simulink library "Power_Ideal2Motor"  (R2020a)
settings: Solver=VariableStepAuto  StartTime=0.0  StopTime=10.0  RelTol=1e-3
undefined symbols (not defined in the file): ShaftF, ShaftR
libraries: fl_lib x11, nesl_utility x6, sm_lib x1
Description:
  | Component of Simscape Vehicle Templates Library
  | 
  | Copyright 2018-2020 The MathWorks, Inc.
settings Model: Creator=smiller  LastModifiedBy=smiller
settings DataIOCC: ReturnWorkspaceOutputs=off
settings DebuggingCC: ArithmeticOperatorsInVariantConditions=warning
settings SFSimCC: CustomCodeUndefinedFunction=UseInterfaceOnly

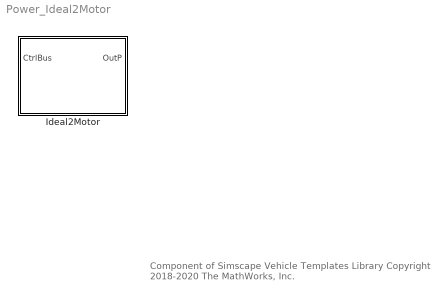
== system Power_Ideal2Motor ==
  note: Component of Simscape Vehicle Templates Library
      | Copyright 2018-2020 The MathWorks, Inc.
  Ideal2Motor : Subsystem  VariantControl=IdealTwoMotor  mask(Two Ideal Motors){motor_ts_f=100, motor_ts_r=100}
      mask prompts: motor_ts_f "Front Motor Cutoff Frequency (Hz)"; motor_ts_r "Rear Motor Cutoff Frequency (Hz)"
      mask Display: image('sm_car_vehicle_power_ideal2motor_IMAGE.png');

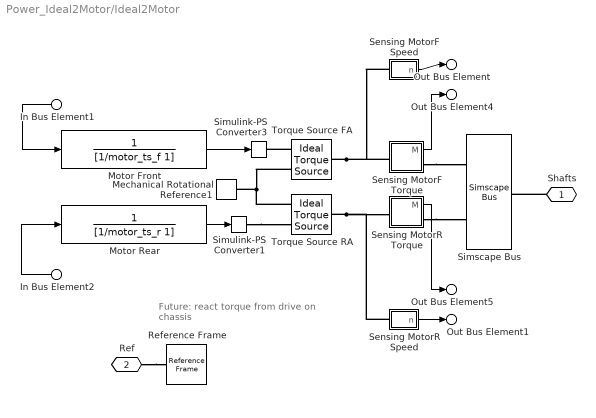
== system Power_Ideal2Motor/Ideal2Motor ==
  note: Future: react torque from
      | drive on chassis
  In Bus Element1 : Inport  PortName=CtrlBus  Element=MMotorFDemand
  In Bus Element2 : Inport  PortName=CtrlBus  Element=MMotorRDemand
  Mechanical Rotational Reference1 : fl_lib/Mechanical/Rotational Elements/Mechanical Rotational Reference
  Motor Front : TransferFcn  Denominator=[1/motor_ts_f 1]
  Motor Rear : TransferFcn  Denominator=[1/motor_ts_r 1]
  Reference Frame : sm_lib/Frames and Transforms/Reference Frame
  Sensing MotorF Speed : Subsystem
  Sensing MotorF Torque : Subsystem
  Sensing MotorR Speed : Subsystem
  Sensing MotorR Torque : Subsystem
  Simscape Bus : SimscapeBus  HierarchyStrings=ShaftF;ShaftR
  Simulink-PS Converter1 : nesl_utility/Simulink-PS Converter  PhysicalDomain=network_engine_domain  SubClassName=ps_input  LeftPortType=input  RightPortType=output  PseudoPeriodic=off  Frequencies=[]  NoiseDistribution=none  NoiseParameters=[]  Unit=1  AffineConversion=off  FilteringAndDerivatives=provide  SimscapeFilterOrder=1  InputFilterTimeConstant=0.001  UdotUserProvided=0
  Simulink-PS Converter3 : nesl_utility/Simulink-PS Converter  PhysicalDomain=network_engine_domain  SubClassName=ps_input  LeftPortType=input  RightPortType=output  PseudoPeriodic=off  Frequencies=[]  NoiseDistribution=none  NoiseParameters=[]  Unit=1  AffineConversion=off  FilteringAndDerivatives=provide  SimscapeFilterOrder=1  InputFilterTimeConstant=0.001  UdotUserProvided=0
  Torque Source FA : fl_lib/Mechanical/Mechanical Sources/Ideal Torque Source
  Torque Source RA : fl_lib/Mechanical/Mechanical Sources/Ideal Torque Source
  Shafts : PMIOPort  Side=Left
  Ref : PMIOPort  Port=2  Side=Right
  Out Bus Element : Outport  VectorParamsAs1DForOutWhenUnconnected=off  PortName=OutP  Element=nMotorF
  Out Bus Element1 : Outport  VectorParamsAs1DForOutWhenUnconnected=off  PortName=OutP  Element=nMotorR
  Out Bus Element4 : Outport  VectorParamsAs1DForOutWhenUnconnected=off  PortName=OutP  Element=MMotorF
  Out Bus Element5 : Outport  VectorParamsAs1DForOutWhenUnconnected=off  PortName=OutP  Element=MMotorR
  wires:
  Sensing MotorR Torque/1(M) -> Out Bus Element5/1
  Sensing MotorF Torque/1(M) -> Out Bus Element4/1
  Motor Rear/1 -> Simulink-PS Converter1/1
  Motor Front/1 -> Simulink-PS Converter3/1
  In Bus Element1/1 -> Motor Front/1
  In Bus Element2/1 -> Motor Rear/1
  Sensing MotorF Speed/1(n) -> Out Bus Element/1
  Sensing MotorR Speed/1(n) -> Out Bus Element1/1
  connections:
  Sensing MotorR Torque/RConn1 -- Simscape Bus/LConn2
  Sensing MotorF Torque/RConn1 -- Simscape Bus/LConn1
  Ref/RConn1 -- Reference Frame/RConn1
  Shafts/RConn1 -- Simscape Bus/RConn1
  Torque Source RA/RConn2 -- Mechanical Rotational Reference1/LConn1 -- Torque Source FA/RConn2
  Simulink-PS Converter1/RConn1 -- Torque Source RA/RConn1
  Torque Source FA/RConn1 -- Simulink-PS Converter3/RConn1
  Torque Source FA/LConn1 -- Sensing MotorF Torque/LConn1 -- Sensing MotorF Speed/LConn1
  Torque Source RA/LConn1 -- Sensing MotorR Torque/LConn1 -- Sensing MotorR Speed/LConn1

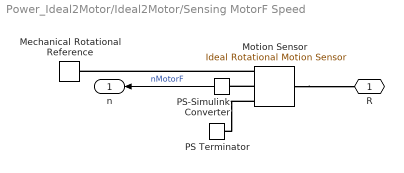
== system Power_Ideal2Motor/Ideal2Motor/Sensing MotorF Speed ==
  Mechanical Rotational Reference : fl_lib/Mechanical/Rotational Elements/Mechanical Rotational Reference
  Motion Sensor : fl_lib/Mechanical/Mechanical Sensors/Ideal Rotational Motion Sensor  wrap_angle=simscape.enum.onoff.off  offset=0 rad
  PS Terminator : fl_lib/Physical Signals/Sinks/PS Terminator
  PS-Simulink Converter : nesl_utility/PS-Simulink Converter  PhysicalDomain=network_engine_domain  SubClassName=ps_output  LeftPortType=input  RightPortType=output  PseudoPeriodic=off  Frequencies=[]  Unit=rad/s  AffineConversion=off
  R : PMIOPort  Side=Left
  n : Outport  VectorParamsAs1DForOutWhenUnconnected=off
  wires:
  PS-Simulink Converter/1 -> n/1  "nMotorF"
  connections:
  Motion Sensor/RConn1 -- Mechanical Rotational Reference/LConn1
  Motion Sensor/LConn1 -- R/RConn1
  Motion Sensor/RConn3 -- PS Terminator/LConn1
  Motion Sensor/RConn2 -- PS-Simulink Converter/LConn1

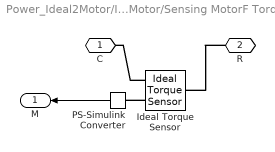
== system Power_Ideal2Motor/Ideal2Motor/Sensing MotorF Torque ==
  Ideal Torque Sensor : fl_lib/Mechanical/Mechanical Sensors/Ideal Torque Sensor
  PS-Simulink Converter : nesl_utility/PS-Simulink Converter  PhysicalDomain=network_engine_domain  SubClassName=ps_output  LeftPortType=input  RightPortType=output  PseudoPeriodic=off  Frequencies=[]  Unit=N*m  AffineConversion=off
  C : PMIOPort  Side=Right
  R : PMIOPort  Port=2  Side=Left
  M : Outport  VectorParamsAs1DForOutWhenUnconnected=off
  wires:
  PS-Simulink Converter/1 -> M/1
  connections:
  Ideal Torque Sensor/RConn1 -- C/RConn1
  R/RConn1 -- Ideal Torque Sensor/LConn1
  Ideal Torque Sensor/RConn2 -- PS-Simulink Converter/LConn1

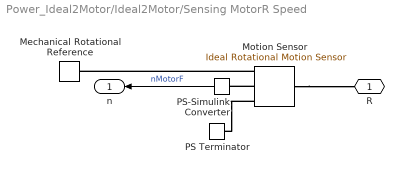
== system Power_Ideal2Motor/Ideal2Motor/Sensing MotorR Speed ==
  Mechanical Rotational Reference : fl_lib/Mechanical/Rotational Elements/Mechanical Rotational Reference
  Motion Sensor : fl_lib/Mechanical/Mechanical Sensors/Ideal Rotational Motion Sensor  wrap_angle=simscape.enum.onoff.off  offset=0 rad
  PS Terminator : fl_lib/Physical Signals/Sinks/PS Terminator
  PS-Simulink Converter : nesl_utility/PS-Simulink Converter  PhysicalDomain=network_engine_domain  SubClassName=ps_output  LeftPortType=input  RightPortType=output  PseudoPeriodic=off  Frequencies=[]  Unit=rad/s  AffineConversion=off
  R : PMIOPort  Side=Left
  n : Outport  VectorParamsAs1DForOutWhenUnconnected=off
  wires:
  PS-Simulink Converter/1 -> n/1  "nMotorF"
  connections:
  Motion Sensor/RConn2 -- PS-Simulink Converter/LConn1
  Motion Sensor/RConn3 -- PS Terminator/LConn1
  Motion Sensor/LConn1 -- R/RConn1
  Motion Sensor/RConn1 -- Mechanical Rotational Reference/LConn1

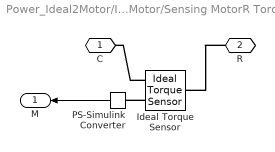
== system Power_Ideal2Motor/Ideal2Motor/Sensing MotorR Torque ==
  Ideal Torque Sensor : fl_lib/Mechanical/Mechanical Sensors/Ideal Torque Sensor
  PS-Simulink Converter : nesl_utility/PS-Simulink Converter  PhysicalDomain=network_engine_domain  SubClassName=ps_output  LeftPortType=input  RightPortType=output  PseudoPeriodic=off  Frequencies=[]  Unit=N*m  AffineConversion=off
  C : PMIOPort  Side=Right
  R : PMIOPort  Port=2  Side=Left
  M : Outport  VectorParamsAs1DForOutWhenUnconnected=off
  wires:
  PS-Simulink Converter/1 -> M/1
  connections:
  Ideal Torque Sensor/RConn2 -- PS-Simulink Converter/LConn1
  R/RConn1 -- Ideal Torque Sensor/LConn1
  Ideal Torque Sensor/RConn1 -- C/RConn1
